simulink model "HoverboardGNCApp"  (R2021b)
settings: Solver=FixedStepAuto  StartTime=0.0  StopTime=inf  RelTol=1e-3
libraries: androiduilib x7, androidcommunicationlib x4, androidsensorlib x3, simulink x1
settings Model: Creator=Admin  LastModifiedBy=Wael
settings OptimizationCC: EnhancedBackFolding=on  PassReuseOutputArgsAs=Individual arguments  ZeroExternalMemoryAtStartup=off  ZeroInternalMemoryAtStartup=off  MaxStackSize=64  OptimizeBlockOrder=speed  DifferentSizesBufferReuse=on  OptimizationCustomize=off  EfficientTunableParamExpr=on
settings DebuggingCC: ParameterTunabilityLossMsg=error
settings HardwareCC: ProdBitPerPointer=32  ProdBitPerSizeT=32  ProdBitPerPtrDiffT=32  ProdLargestAtomicInteger=Long  ProdLargestAtomicFloat=Double  ProdWordSize=32  ProdHWDeviceType=ARM Compatible->ARM Cortex
settings SFSimCC: MATLABDynamicMemAlloc=off
settings RTWCC: Description=Embedded Coder  SystemTargetFile=ert.tlc  HardwareBoard=Android Device  TLCOptions="-aInlineSetEventsForThisBaseRateFcn=TLC_FALSE -aSuppressMultiTaskScheduler=TLC_FALSE  -aRateBasedStepFcn=0"  TemplateMakefile=ert_default_tmf  RTWVerbose=off  Toolchain=Android SDK/NDK Tools
settings CodeAppCC: ForceParamTrailComments=on  IgnoreCustomStorageClasses=off  OperatorAnnotations=on  SimulinkDataObjDesc=on  SFDataObjDesc=on  InsertBlockDesc=on
settings ERTTargetCC: SupportVariableSizeSignals=on

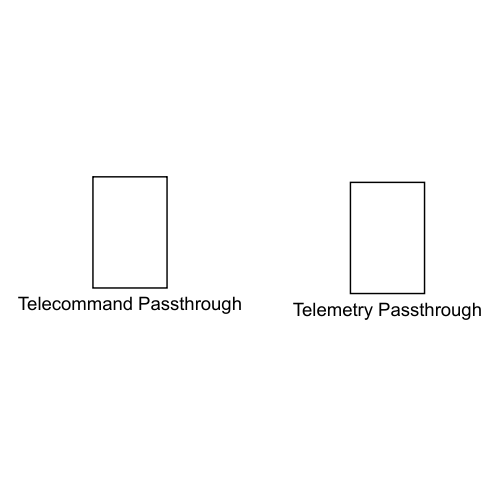
[thumbnail: Simulink's stored preview of the top-level diagram]
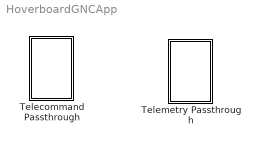
== system HoverboardGNCApp ==
  Telecommand Passthrough : Subsystem
  Telemetry Passthrough : Subsystem

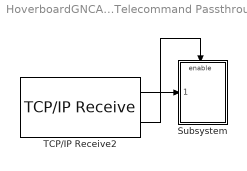
== system HoverboardGNCApp/Telecommand Passthrough ==
  Subsystem : Subsystem
  TCP/IP Receive2 : androidcommunicationlib/TCP//IP Receive  TCPReceiveId=HoverboardGNC25/Telecommand_Passthrough/TCP//IP_Receive2  Mode_=Server  LocalServerPort_=25000  RemoteAddr_=192.168.1.2  RemoteServerPort_=8000  DataType_=uint8  DataSize_=8  SampleTime_=0.1  ClientPortBindingSelection_=off  ClientPortToBind_=35000  BlockingMode_=off  BlockTimeout_=0.1
      settings: SourceProductBaseCode=ANDROID
  wires:
  TCP/IP Receive2/2 -> Subsystem/Enable
  TCP/IP Receive2/1 -> Subsystem/1(buffer_in)

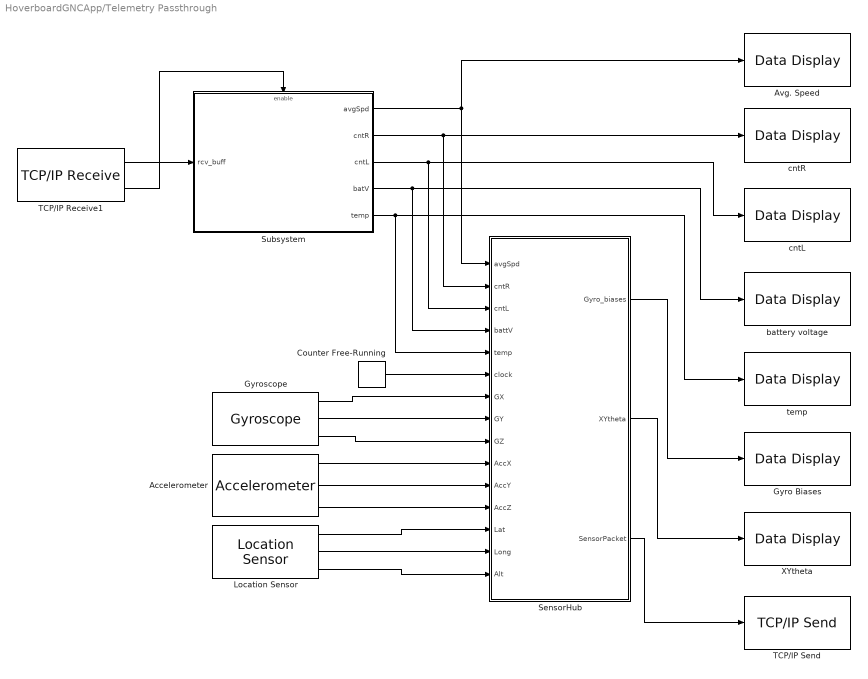
== system HoverboardGNCApp/Telemetry Passthrough ==
  Accelerometer : androidsensorlib/Accelerometer  OutputVector=off  SampleTime=0.1  BlockPlatform=Android
      settings: SourceProductBaseCode=ANDROID
  Avg. Speed : androiduilib/Data Display  DataDisplayId=HoverboardGNC25/Telemetry_Passthrough/Avg._Speed  Format=Float  Precision=6  SimulateUsing=Code generation  blockPlatform=Android
      settings: SourceProductBaseCode=ANDROID
  Counter Free-Running : simulink/Sources/Counter Free-Running  NumBits=16  tsamp=0.1
  Gyro Biases : androiduilib/Data Display  DataDisplayId=HoverboardGNC25/Telemetry_Passthrough/Gyro_Biases  Format=Float  Precision=6  SimulateUsing=Code generation  blockPlatform=Android
      settings: SourceProductBaseCode=ANDROID
  Gyroscope : androidsensorlib/Gyroscope  OutputVector=off  SampleTime=0.1  BlockPlatform=Android
      settings: SourceProductBaseCode=ANDROID
  Location Sensor : androidsensorlib/Location Sensor  OutputVector=off  SampleTime=0.1  BlockPlatform=Android
      settings: SourceProductBaseCode=ANDROID
  SensorHub : MATLAB Function  TreatAsAtomicUnit=on
  Subsystem : Subsystem
  TCP/IP Receive1 : androidcommunicationlib/TCP//IP Receive  TCPReceiveId=HoverboardGNC25/Telemetry_Passthrough/TCP//IP_Receive1  Mode_=Client  LocalServerPort_=25000  RemoteAddr_=192.168.1.2  RemoteServerPort_=8000  DataType_=uint8  DataSize_=22  SampleTime_=0.1  ClientPortBindingSelection_=off  ClientPortToBind_=35000  BlockingMode_=off  BlockTimeout_=0.1
      settings: SourceProductBaseCode=ANDROID
  TCP/IP Send : androidcommunicationlib/TCP//IP Send  TCPSendId=HoverboardGNC25/Telemetry_Passthrough/TCP//IP_Send  Mode_=Server  LocalServerPort_=25000  RemoteAddr_=127.0.0.1  RemoteServerPort_=25000  ClientPortBindingSelection_=off  ClientPortToBind_=35000  BlockingMode_=off  BlockTimeout_=0.1
      settings: SourceProductBaseCode=ANDROID
  XYtheta : androiduilib/Data Display  DataDisplayId=HoverboardGNC25/Telemetry_Passthrough/XYtheta  Format=Float  Precision=6  SimulateUsing=Code generation  blockPlatform=Android
      settings: SourceProductBaseCode=ANDROID
  battery voltage : androiduilib/Data Display  DataDisplayId=HoverboardGNC25/Telemetry_Passthrough/battery_voltage  Format=Float  Precision=6  SimulateUsing=Code generation  blockPlatform=Android
      settings: SourceProductBaseCode=ANDROID
  cntL : androiduilib/Data Display  DataDisplayId=HoverboardGNC25/Telemetry_Passthrough/cntL  Format=Float  Precision=6  SimulateUsing=Code generation  blockPlatform=Android
      settings: SourceProductBaseCode=ANDROID
  cntR : androiduilib/Data Display  DataDisplayId=HoverboardGNC25/Telemetry_Passthrough/cntR  Format=Float  Precision=6  SimulateUsing=Code generation  blockPlatform=Android
      settings: SourceProductBaseCode=ANDROID
  temp : androiduilib/Data Display  DataDisplayId=HoverboardGNC25/Telemetry_Passthrough/temp  Format=Float  Precision=6  SimulateUsing=Code generation  blockPlatform=Android
      settings: SourceProductBaseCode=ANDROID
  wires:
  Gyroscope/2 -> SensorHub/8(GY)
  Gyroscope/3 -> SensorHub/9(GZ)
  Accelerometer/2 -> SensorHub/11(AccY)
  Gyroscope/1 -> SensorHub/7(GX)
  Accelerometer/3 -> SensorHub/12(AccZ)
  Accelerometer/1 -> SensorHub/10(AccX)
  Counter Free-Running/1 -> SensorHub/6(clock)
  Location Sensor/1 -> SensorHub/13(Lat)
  Location Sensor/2 -> SensorHub/14(Long)
  Location Sensor/3 -> SensorHub/15(Alt)
  SensorHub/1(Gyro_biases) -> Gyro Biases/1
  SensorHub/3(SensorPacket) -> TCP/IP Send/1
  SensorHub/2(XYtheta) -> XYtheta/1
  Subsystem/1(avgSpd) -> SensorHub/1(avgSpd), Avg. Speed/1
  Subsystem/2(cntR) -> SensorHub/2(cntR), cntR/1
  Subsystem/3(cntL) -> SensorHub/3(cntL), cntL/1
  Subsystem/4(batV) -> SensorHub/4(battV), battery voltage/1
  TCP/IP Receive1/2 -> Subsystem/Enable
  TCP/IP Receive1/1 -> Subsystem/1(rcv_buff)
  Subsystem/5(temp) -> SensorHub/5(temp), temp/1

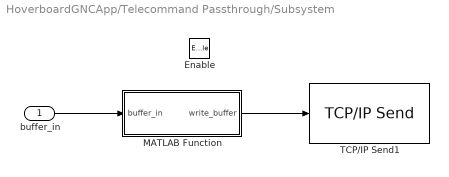
== system HoverboardGNCApp/Telecommand Passthrough/Subsystem ==
  buffer_in : Inport
  Enable : EnablePort
  MATLAB Function : MATLAB Function  TreatAsAtomicUnit=on
  TCP/IP Send1 : androidcommunicationlib/TCP//IP Send  TCPSendId=HoverboardGNC25/Telecommand_Passthrough/Subsystem/TCP//IP_Send1  Mode_=Client  LocalServerPort_=25000  RemoteAddr_=192.168.1.2  RemoteServerPort_=8000  ClientPortBindingSelection_=off  ClientPortToBind_=35000  BlockingMode_=off  BlockTimeout_=0.1
      settings: SourceProductBaseCode=ANDROID
  wires:
  MATLAB Function/1(write_buffer) -> TCP/IP Send1/1
  buffer_in/1 -> MATLAB Function/1(buffer_in)

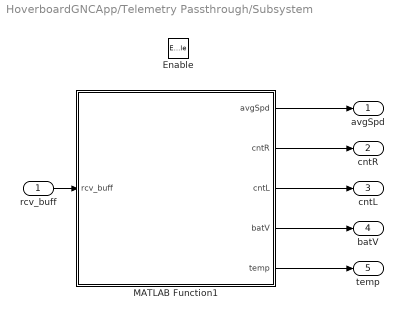
== system HoverboardGNCApp/Telemetry Passthrough/Subsystem ==
  rcv_buff : Inport
  Enable : EnablePort
  MATLAB Function1 : MATLAB Function  TreatAsAtomicUnit=on
  avgSpd : Outport
  cntR : Outport  Port=2
  cntL : Outport  Port=3
  batV : Outport  Port=4
  temp : Outport  Port=5
  wires:
  MATLAB Function1/3(cntL) -> cntL/1
  MATLAB Function1/4(batV) -> batV/1
  MATLAB Function1/2(cntR) -> cntR/1
  MATLAB Function1/5(temp) -> temp/1
  rcv_buff/1 -> MATLAB Function1/1(rcv_buff)
  MATLAB Function1/1(avgSpd) -> avgSpd/1

== matlab function HoverboardGNCApp/Telemetry Passthrough/Subsystem/MATLAB Function1 ==
  data: avgSpd output size=1; cntR output int16 size=1; cntL output int16 size=1; batV output single size=1; rcv_buff input; temp output single size=1
function [avgSpd, cntR, cntL, batV, temp]  = fcn(rcv_buff)
% header = rvc_buff(1:2);
% cmd1 = rvc_buff(3:4);
% cmd2 = rvc_buff(5:6);
% cmdLED = rvc_buff(19:20);
% chkSum = rvc_buff(21:22);
% 

spdR = typecast(rcv_buff(7:8) , 'int16');
spdL = typecast(rcv_buff(9:10) , 'int16');
if(spdR>32767)
    spdR = spdR-65536;
end
if(spdL>32767)
    spdL = spdL-65536;
end
% avgSpd = (double(spdR)+double(spdL))*0.5;
avgSpd = double(spdR);


cntR = typecast(rcv_buff(11:12) , 'int16');
cntL = typecast(rcv_buff(13:14) , 'int16');

batV = single(typecast(rcv_buff(15:16) , 'int16'))/100;

temp = single(typecast(rcv_buff(17:18) , 'int16'))/10;

end

== matlab function HoverboardGNCApp/Telecommand Passthrough/Subsystem/MATLAB Function ==
  data: write_buffer output size=[1 8]; buffer_in input uint8
function write_buffer  = fcn(buffer_in)

steer = typecast((buffer_in(3:4)),'uint16');
speed = typecast((buffer_in(5:6)),'uint16');

start = uint16(43981);
steerp = uint16(steer);
speedp = uint16(speed);
chkSum = bitxor(bitxor(start,steerp),speedp);
chkSum = typecast((chkSum),'uint16');
write_buffer = [typecast((start),'uint8'),typecast((steerp),'uint8'),typecast((speedp),'uint8'),typecast((chkSum),'uint8')];


% Hoverboard Diameter = 0.1651 m
% m/s -> rpm : 60/(0.1651*pi) = x 115.68
% k = -1;  %Scaling factor to account for wheel balancing, negative for orientation wrt robot body
% scale = 115.68*k;
% speed = scale * TwistMsg.Linear.X;
% steer = scale * TwistMsg.Angular.Z;
% 
% % RPM Range = [-550 550], Approx. Speed Range = [-17 17] KPH (measured
% % without load). Should limit to a lower value to prevent accidents
%

== matlab function HoverboardGNCApp/Telemetry Passthrough/SensorHub ==
  data: Gyro_biases output; XYtheta output; avgSpd input; cntR input; cntL input; battV input; temp input; SensorPacket output uint8 size=[1 12]; clock input; GX input; GY input; GZ input; AccX input; AccY input; AccZ input; Lat input; Long input; Alt input
function [Gyro_biases,XYtheta,SensorPacket]  = AccGyrFusion(avgSpd, cntR, cntL, battV, temp, clock, GX, GY, GZ, AccX, AccY, AccZ, Lat, Long, Alt)
%Some phones's gyros have more drift than others. Xiaomi RedNote 8 pro is
%quite stable. Honor 7 not so much. Calibrate by finding the gyro bias when
%still. Honor 7 drifts by as much as 1.4 degrees in a minute. With biases
%estimated during first 3 seconds, it drifts by 0.15 degrees roughly in a
%minute. 
persistent yaw;
persistent pitch;
persistent roll;
persistent biases;
persistent cntRprev;
persistent cntLprev;
persistent PosX;
persistent PosY;
persistent GPS_lat_prev;
persistent GPS_lon_prev;

% --------------------------------------------------------------
% 0- Initialize
% --------------------------------------------------------------

if(isempty(yaw))
    yaw = double(0);
    pitch = double(0);
    roll = double(0);
    biases = [GX,GY,GZ];
    cntRprev = double(cntR);
    cntLprev = double(cntL);    
    PosX = double(Long);
    PosY = double(Lat);    
    GPS_lat_prev = PosY;
    GPS_lon_prev = PosX;
end

% --------------------------------------------------------------
% 1- Fuse Accelerometer & Gyroscope to get orientation 
% --------------------------------------------------------------
g = sqrt(AccX^2 + AccY^2 + AccZ^2);
if(g<0.01)
    g = single(9.8);
end
Acc_pitch = double(asin(AccX/g));
Acc_roll = double(atan2(AccY,AccZ));

if(clock<50)
    biases = biases*0.99 + [GX,GY,GZ]*0.01;
end
Gyro_biases = biases;

GX = GX-biases(1);
GY = GY-biases(2);
GZ = GZ-biases(3);
%Rotate Gyro sensor frame to world frame
GX_w = GX + GY*sin(roll)*tan(pitch) + GZ*cos(roll)*tan(pitch);
GY_w = GY*cos(roll) - GZ*sin(roll);
GZ_w = GY*sin(roll)/cos(pitch) + GZ*cos(roll)/cos(pitch);

dt = double(0.1);
alpha = double(0.05);

if(~isnan(GX_w))
    roll = roll + double(GX_w)*dt;
    roll = roll*(1-alpha) + Acc_roll*alpha;
    roll = wrapToPi(roll);
end

if(~isnan(GY_w))
    pitch = pitch + double(GY_w)*dt;
    pitch = pitch*(1-alpha) + Acc_pitch*alpha;
    pitch = wrapToPi(pitch);
end

if(~isnan(GZ_w))
    yaw = yaw + double(GZ_w)*dt;
    yaw = wrapToPi(yaw);
end

% --------------------------------------------------------------
% 2- Calculate position based on wheel encoder data
% --------------------------------------------------------------
% Take care of the roll over in wheel encoder values
dR = double(cntR) - cntRprev;
if(dR<-4500)
    dR = dR + 9000;
end
if(dR>4500)
    dR = dR - 9000;
end
dL = double(cntL) - cntLprev;
if(dL<-4500)
    dL = dL + 9000;
end
if(dL>4500)
    dL = dL - 9000;
end
cntRprev = double(cntR);
cntLprev = double(cntL);
% % wheel encoders approx. 90 counts per rev
% % rev -> m : scale_dist = (0.1651*pi)/90 = 0.005763
% %Scaling factor to be adjusted to account for wheel balancing, negative for orientation wrt robot body
scale_dist = 0.00594;
meanD = (dR+dL)*0.5*scale_dist;
Sc_lat = 111194.9266445882; %Scales for Jeddah. found using getDistanceBearing func.
Sc_lon = 103460.3604049077;
PosX = PosX + meanD*cos(yaw)/Sc_lon;
PosY = PosY + meanD*sin(yaw)/Sc_lat;

% --------------------------------------------------------------
% 3- Apply GPS update to XYtheta
% --------------------------------------------------------------

[R,GPSheading] = getDistanceBearing([GPS_lat_prev,GPS_lon_prev],[Lat,Long],1);
if(R>0.001)
    PosX = PosX*0.99 + Long*0.01;
    PosY = PosY*0.99 + Lat*0.01;
    GPS_lat_prev = Lat;
    GPS_lon_prev = Long;
    if(avgSpd<-30)%Do GPS-based orientation update only when moving
        yaw = fuseAngles(yaw,GPSheading,0.95);
    end
end

% Signs and order of yaw pitch roll changed to correspond to ROS conventions.
% SensorPacket = [typecast(single(yaw),'uint8'),typecast(single(-roll),'uint8'),typecast(single(pitch),'uint8'),typecast(single(PosX),'uint8'),typecast(single(PosY),'uint8'),typecast(single(Lat),'uint8'),typecast(single(Long),'uint8'),typecast(cntR,'uint8'),typecast(cntL,'uint8'),typecast(single(AccX),'uint8'),typecast(single(AccY),'uint8'),typecast(single(AccZ),'uint8'),typecast(single(GX),'uint8'),typecast(single(GY),'uint8'),typecast(single(GZ),'uint8'),typecast(single(battV),'uint8'),typecast(single(temp),'uint8')];
%64
SensorPacket = [typecast(single(yaw),'uint8'),typecast(single(PosX),'uint8'),typecast(single(PosY),'uint8')];
%12
% SensorPacket = [typecast(single(yaw),'uint8'),typecast(single(PosX),'uint8'),typecast(single(PosY),'uint8'),typecast(single(Lat),'uint8'),typecast(single(Long),'uint8')];
%20
XYtheta = [PosY,PosX,yaw*180/pi];
end
